simulink model "tc387_xcp_stim_demo"  (R2026a)
settings: Solver=FixedStepDiscrete  StopTime=5.0  FixedStep=0.001
undefined symbols (not defined in the file): FOC_20kHz, g_foc_exec_time_us, g_foc_isr_counter, g_hil_curr_u, g_hil_mode_enable, g_meas_curr_u
libraries: xcpprotocollib x3
settings Model: Creator=probst  LastModifiedBy=probst

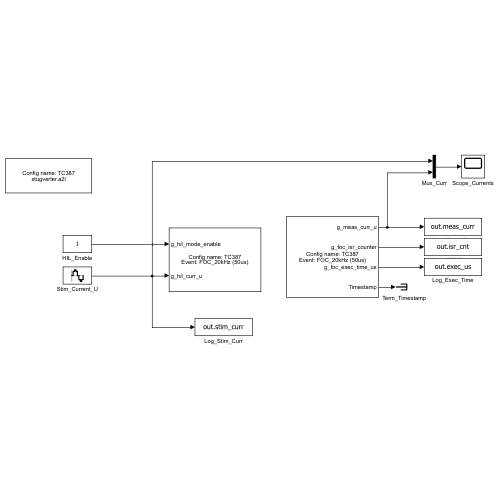
[thumbnail: Simulink's stored preview of the top-level diagram]
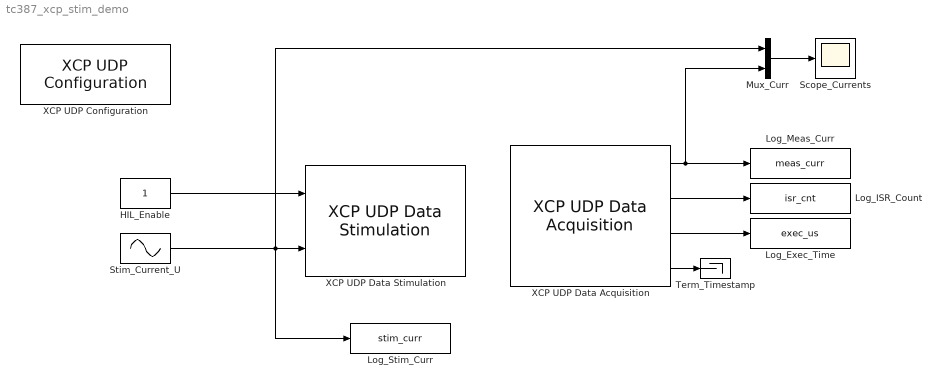
== system tc387_xcp_stim_demo ==
  HIL_Enable : Constant  OutDataTypeStr=double  SampleTime=0.001
  Log_Exec_Time : ToWorkspace  VariableName=exec_us  SaveFormat=Timeseries  SampleTime=-1
  Log_ISR_Count : ToWorkspace  VariableName=isr_cnt  SaveFormat=Timeseries  SampleTime=-1
  Log_Meas_Curr : ToWorkspace  VariableName=meas_curr  SaveFormat=Timeseries  SampleTime=-1
  Log_Stim_Curr : ToWorkspace  VariableName=stim_curr  SaveFormat=Timeseries  SampleTime=-1
  Mux_Curr : Mux  Inputs=2
  Scope_Currents : Scope
      settings: ActiveDisplayYMinimum=-37.5  ActiveDisplayYMaximum=37.5
  Stim_Current_U : Sin  Amplitude=30.0  Frequency=2*pi*2.0  SampleTime=0.001
  Term_Timestamp : Terminator
  XCP UDP Configuration : xcpprotocollib/UDP/XCP UDP Configuration  Priority=-100  SlaveName=TC387  SlaveID=1  A2LFile=C:\Users\probst\Desktop\stugverter\simulink\scripts\..\..\firmware\stugverter.a2l  EnableSecurity=off  ConnectMode=off  EnableStatus=off  SampleTime=0.001  HeaderErrDet=on  CTRScheme=One counter for all CTOs and DTOs  LocalAddress=auto  LocalPort=auto  DAQTimeout=Inf
      settings: LibrarySourceBlock=vntxcplib/UDP/XCP UDP Configuration
  XCP UDP Data Acquisition : xcpprotocollib/UDP/XCP UDP Data Acquisition  SlaveName=TC387  A2LFile=C:\Users\probst\Desktop\stugverter\simulink\scripts\..\..\firmware\stugverter.a2l  EventName=FOC_20kHz (50us)  SelectedMeasurements=g_meas_curr_u;g_foc_isr_counter;g_foc_exec_time_us  DAQPriority=0  SampleTime=0.001  EnableTimestamp=on  InputOrOutputDatatype=Raw values as double (no Compu method conversion)
      settings: LibrarySourceBlock=vntxcplib/UDP/XCP UDP Data Acquisition
  XCP UDP Data Stimulation : xcpprotocollib/UDP/XCP UDP Data Stimulation  SlaveName=TC387  A2LFile=C:\Users\probst\Desktop\stugverter\simulink\scripts\..\..\firmware\stugverter.a2l  EventName=FOC_20kHz (50us)  SelectedMeasurements=g_hil_mode_enable;g_hil_curr_u  EnableTimestamp=off  InputOrOutputDatatype=Raw values as double (no Compu method conversion)
      settings: LibrarySourceBlock=vntxcplib/UDP/XCP UDP Data Stimulation
  wires:
  HIL_Enable/1 -> XCP UDP Data Stimulation/1
  Stim_Current_U/1 -> Log_Stim_Curr/1, Mux_Curr/1, XCP UDP Data Stimulation/2
  XCP UDP Data Acquisition/1 -> Log_Meas_Curr/1, Mux_Curr/2
  XCP UDP Data Acquisition/2 -> Log_ISR_Count/1
  XCP UDP Data Acquisition/3 -> Log_Exec_Time/1
  XCP UDP Data Acquisition/4 -> Term_Timestamp/1
  Mux_Curr/1 -> Scope_Currents/1
